simulink model "example_THB_set_T"  (R2013b)
settings: Solver=FixedStepDiscrete  StartTime=0.0  StopTime=10.0  FixedStep=1  RelTol=1e-3
libraries: carnot x2
settings Model: Creator=awohlfei  LastModifiedBy=awohlfei

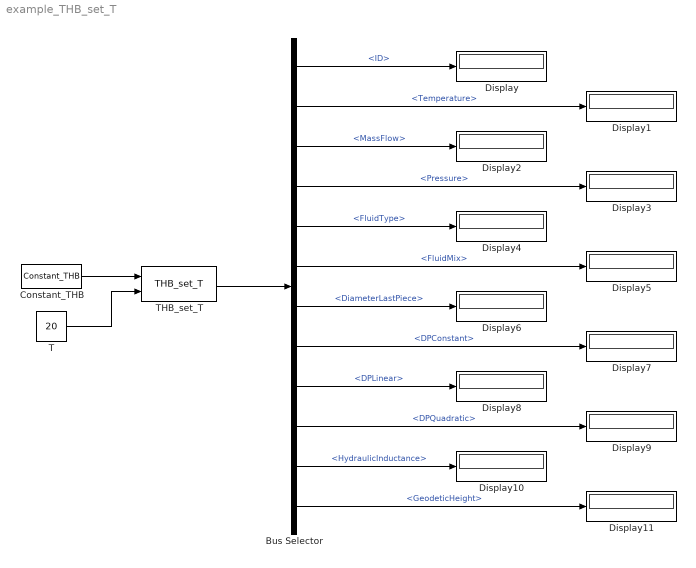
== system example_THB_set_T ==
  Bus Selector : BusSelector  OutputSignals=ID,Temperature,MassFlow,Pressure,FluidType,FluidMix,DiameterLastPiece,DPConstant,DPLinear,DPQuadratic,HydraulicInductance,GeodeticHeight
  Constant_THB : carnot/Source/Simple/Constant_THB  t=40  mdot=0  p=1e5  mID=No Pressure Drop  fluid=Water  mix=0  dia=0.02  hgt=0
  Display{,1..11} (12 alike) : Display
  T : Constant  Value=20
  THB_set_T : carnot/Source/Simple/THB_set_T
  wires:
  Constant_THB/1 -> THB_set_T/1
  THB_set_T/1 -> Bus Selector/1
  T/1 -> THB_set_T/2
  Bus Selector/1 -> Display/1  "<ID>"
  Bus Selector/2 -> Display1/1  "<Temperature>"
  Bus Selector/3 -> Display2/1  "<MassFlow>"
  Bus Selector/4 -> Display3/1  "<Pressure>"
  Bus Selector/5 -> Display4/1  "<FluidType>"
  Bus Selector/6 -> Display5/1  "<FluidMix>"
  Bus Selector/7 -> Display6/1  "<DiameterLastPiece>"
  Bus Selector/8 -> Display7/1  "<DPConstant>"
  Bus Selector/9 -> Display8/1  "<DPLinear>"
  Bus Selector/10 -> Display9/1  "<DPQuadratic>"
  Bus Selector/11 -> Display10/1  "<HydraulicInductance>"
  Bus Selector/12 -> Display11/1  "<GeodeticHeight>"
